simulink model "model"  (R2020b)
settings: Solver=FixedStepAuto  StartTime=0.0  StopTime=10.0  FixedStep=0.1e-4  RelTol=1e-3
model workspace (MAT data in the model file):
  a = -41900
  b = -1.22
  c = 2.44e-05
  d = 0.000588
settings Model: OrderedModelArguments=off  Creator=Pavan  LastModifiedBy=Pavan

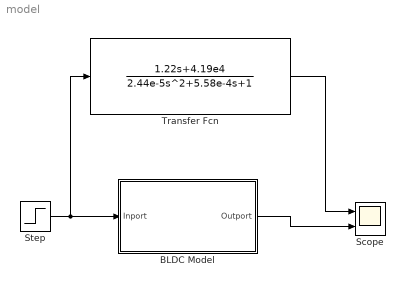
== system model ==
  BLDC Model : Subsystem
  Scope : Scope  NumInputPorts=2
  Step : Step  Time=0  After=2000  SampleTime=0
  Transfer Fcn : TransferFcn  Numerator=[1.22 4.19e4]  Denominator=[2.44e-5 5.58e-4 1]
  wires:
  Step/1 -> BLDC Model/1(Inport), Transfer Fcn/1
  BLDC Model/1(Outport) -> Scope/2
  Transfer Fcn/1 -> Scope/1

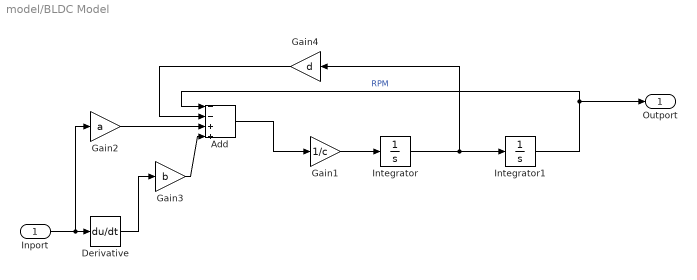
== system model/BLDC Model ==
  Inport : Inport
  Add : Sum  Inputs=--++
  Derivative : Derivative
  Gain1 : Gain  Gain=1/c
  Gain2 : Gain  Gain=a
  Gain3 : Gain  Gain=b
  Gain4 : Gain  Gain=d
  Integrator : Integrator
  Integrator1 : Integrator
  Outport : Outport
  wires:
  Gain4/1 -> Add/2
  Derivative/1 -> Gain3/1
  Inport/1 -> Gain2/1, Derivative/1
  Gain2/1 -> Add/3
  Gain3/1 -> Add/4
  Integrator1/1 -> Outport/1, Add/1  "RPM"
  Integrator/1 -> Gain4/1, Integrator1/1
  Gain1/1 -> Integrator/1
  Add/1 -> Gain1/1
